simulink model "controlGPI_pos_3dof_conMI"  (R2023b)
settings: Solver=VariableStepAuto  StartTime=0.0  StopTime=tsim  FixedStep=1e-5  MaxStep=tstep  RelTol=1e-3
undefined symbols (not defined in the file): contr_robot_params, ddq, dq, MI_Contr1, MI_Contr2, MI_Contr3, MI_motor1, MI_motor2, MI_motor3, ndof, NN_Bspline_params, NN_RBF_params, nn_select, ns, Pc, q, q0, q_cero, q_eq, robot_params, sigbuilder_block, t_qeq_init, t_tr_init, t_trtr, tau_L, tau_L_mags, tr_muestra, Wc, Zc
libraries: mcbcontrolslib x6, spsRMSLib x6, simulink x2
(part 3 of 3)

== matlab function controlGPI_pos_3dof_conMI/Actuadores (Motores de inducción)/MI1 + PBC Torque Controller/Controlador PBC/Ley de control/Ley de control ==
  data: MI_motor_params input; i_Sref input size=[2,1]; d_iSref input size=[2,1]; U_S output size=[2 1]; psi_Rref input size=[2,1]; w_R input; e_Is input; KI_s input
function U_S = fcn(MI_motor_params,i_Sref,d_iSref,psi_Rref,w_R,e_Is,KI_s)

R_R = MI_motor_params.elecparams.R_R;
L_R = MI_motor_params.elecparams.L_R;
M = MI_motor_params.elecparams.M;
n_p = MI_motor_params.elecparams.n_p;

sigma = MI_motor_params.elecparams.sigma;
gamma = MI_motor_params.elecparams.gamma;

dI_Saref = d_iSref(1);
dI_Sbref = d_iSref(2);

I_Saref = i_Sref(1);
I_Sbref = i_Sref(2);

psi_Raref = psi_Rref(1);
psi_Rbref = psi_Rref(2);

e_ISa = e_Is(1);
e_ISb = e_Is(2);

U_Sa = sigma*dI_Saref - n_p*M/L_R*w_R*psi_Rbref + sigma*gamma*I_Saref - R_R*M/L_R^2*psi_Raref - KI_s*e_ISa;
U_Sb = sigma*dI_Sbref + n_p*M/L_R*w_R*psi_Raref + sigma*gamma*I_Sbref - R_R*M/L_R^2*psi_Rbref - KI_s*e_ISb;

U_S = [U_Sa;U_Sb];

== matlab function controlGPI_pos_3dof_conMI/Actuadores (Motores de inducción)/MI2 + PBC Torque Controller/Modelo MI (Subsistema eléctrico)/Modelo Motor de inducción (Subsistema eléctrico) ==
  data: MI_motor_params input; di_Sab output double size=[2 1]; dpsi_Rab output double size=[2 1]; u_Sab input double size=[2 1]; i_Sab input double size=[2 1]; psi_Rab input double size=[2 1]; w_R input double size=1; tau_R output size=1; tau_L input
function [di_Sab,dpsi_Rab,tau_R] = fcn(MI_motor_params,u_Sab,i_Sab,psi_Rab,w_R,tau_L)

R_S = MI_motor_params.elecparams.R_S;
R_R = MI_motor_params.elecparams.R_R;
L_S = MI_motor_params.elecparams.L_S;
L_R = MI_motor_params.elecparams.L_R;
M = MI_motor_params.elecparams.M;
n_p = MI_motor_params.elecparams.n_p;

J = MI_motor_params.mechparams.J;
b = MI_motor_params.mechparams.b;

sigma = MI_motor_params.elecparams.sigma;
gamma = MI_motor_params.elecparams.gamma;

u_sa = u_Sab(1);
u_sb = u_Sab(2);

i_sa = i_Sab(1);
i_sb = i_Sab(2);

psi_ra = psi_Rab(1);
psi_rb = psi_Rab(2);

tau_R = n_p*M/L_R*(i_sb*psi_ra-i_sa*psi_rb);

x = [i_sa;i_sb;psi_ra;psi_rb];

A = [-gamma      , 0            , (M*R_R)/(sigma*L_R^2)    , (n_p*M)/(sigma*L_R)*w_R ;
     0           , -gamma       , -(n_p*M)/(sigma*L_R)*w_R , (M*R_R)/(sigma*L_R^2)   ; 
     (R_R*M)/L_R , 0            , -R_R/L_R                 , -n_p*w_R                ;
     0           , (R_R*M)/L_R  , n_p*w_R                  , -R_R/L_R                ];

B = [1/sigma , 0       ;
     0       , 1/sigma ;
     0       , 0       ;
     0       , 0       ];

dx = A*x + B*[u_sa;u_sb];

di_Sab = dx(1:2);
dpsi_Rab = dx(3:4);

%Subsistema mecanico
%dw_R = (1/J)*tau_R - (b/J)*w_R - (1/J)*tau_L;

== matlab function controlGPI_pos_3dof_conMI/ControladorGPI + NN/Matriz D ==
  data: robot_params input Bus: robot_params_bus; robot_din output Bus: robot_din_bus; q input
function robot_din = fcn(robot_params,q)

robot_din = robot_dinm.din_3dof(robot_params,q,zeros(size(q)));

== matlab function controlGPI_pos_3dof_conMI/Perfil torque de carga tau_L/If Action Subsystem/Polinomio 7mo orden sen ==
  data: t input; perfil_params input; qpol output; vpol output; apol output; jpol output
function [qpol,vpol,apol,jpol] = fcn(t,perfil_params)

%Trayectoria de referencia

q0 = 0;
q1 = perfil_params.senoidal.amplitud;

% v0 = perfil_params.polinomio7.vel.inicial;
% v1 = perfil_params.polinomio7.vel.final;
% 
% ac0 = perfil_params.polinomio7.acel.inicial;
% ac1 = perfil_params.polinomio7.acel.final;
% 
% j0 = perfil_params.polinomio7.jerk.inicial;
% j1 = perfil_params.polinomio7.jerk.inicial;

if perfil_params.senoidal.tiempo_inicio-1>0
    t0 = perfil_params.senoidal.tiempo_inicio-1;
else
    t0 = 0;
end
t1 = perfil_params.senoidal.tiempo_inicio;

% Coeficientes de un polinomio de 7mo grado
[qpol,vpol,apol,jpol] = pol7(t,q1,q0,t0,t1);

== matlab function controlGPI_pos_3dof_conMI/Perfil torque de carga tau_L/If Action Subsystem/Senoidal tiempo de inicio ==
  data: t input; tr output; perfil_params input
function tr = fcn(t,perfil_params)

t1 = perfil_params.senoidal.tiempo_inicio;

if t < t1
    tr = 0;
else
    tr = t - t1;
end

== matlab function controlGPI_pos_3dof_conMI/Perfil torque de carga tau_L/If Action Subsystem4/Polinomio 7mo orden tau_L ==
  data: t input; perfil_params input; qpol output; vpol output; apol output; jpol output
function [qpol,vpol,apol,jpol] = fcn(t,perfil_params)

%Trayectoria de referencia

q0 = perfil_params.polinomio7.pos.inicial;
q1 = perfil_params.polinomio7.pos.final;

% v0 = perfil_params.polinomio7.vel.inicial;
% v1 = perfil_params.polinomio7.vel.final;
% 
% ac0 = perfil_params.polinomio7.acel.inicial;
% ac1 = perfil_params.polinomio7.acel.final;
% 
% j0 = perfil_params.polinomio7.jerk.inicial;
% j1 = perfil_params.polinomio7.jerk.inicial;

t0 = perfil_params.polinomio7.tiempo.inicial;
t1 = perfil_params.polinomio7.tiempo.final;

% Coeficientes de un polinomio de 7mo grado
[qpol,vpol,apol,jpol] = pol7(t,q0,q1,t0,t1);

== matlab function controlGPI_pos_3dof_conMI/Actuadores (Motores de inducción)/MI2 + PBC Torque Controller/Modelo MI (Subsistema eléctrico)/ab//dq ==
  data: psi_ra input; psi_Rmag output; psi_rb input; rho output
function [psi_Rmag,rho] = fcn(psi_ra,psi_rb)

psi_Rmag = sqrt(psi_ra^2+psi_rb^2);
rho = atan2(psi_rb,psi_ra);

== matlab function controlGPI_pos_3dof_conMI/Perfil torque de carga tau_L/If Action Subsystem5/Tren de esca ==
  data: t input; q output; perfil_params input
function q = fcn(t,perfil_params)

q = Perfil_trayectoria.trEsca(t,perfil_params);

== matlab function controlGPI_pos_3dof_conMI/Perfil torque de carga tau_L/If Action Subsystem6/Polinomio 7mo orden timeseries ==
  data: t input; qpol output; vpol output; apol output; jpol output
function [qpol,vpol,apol,jpol] = fcn(t)

q0 = 0;
q1 = 1;

t0 = 0.5;
t1 = 1;

%Trayectoria de referencia

% Coeficientes de un polinomio de 7mo grado
[qpol,vpol,apol,jpol] = pol7(t,q0,q1,t0,t1);

== matlab function controlGPI_pos_3dof_conMI/Perfil torque de carga tau_L/If Action Subsystem7/Trayectoria 15 segmentos ==
  data: t input size=1; q output size=1; perfil_params input
function q = fcn(t,perfil_params)

q0 = perfil_params.tr15segs.pos.inicial;
q1 = perfil_params.tr15segs.pos.final;

t0 = perfil_params.tr15segs.tiempo.inicial;

vel_path = perfil_params.tr15segs.vel_path;
acel_path = perfil_params.tr15segs.acel_path;
snap_path = perfil_params.tr15segs.snap_path;

dist = norm(q1-q0);
num_steps = 1000;




[interq,T] = pol15segs.bounded_tr(dist,num_steps,vel_path,acel_path,snap_path,0);

tstep = T/num_steps;
t1 = t0 + T;
t_tr = (t0:tstep:t1)';


[~,idt] = min(t_tr-t);
dire = (q1 - q0)/dist;
q = q0 + dire*interq(idt);

== matlab function controlGPI_pos_3dof_conMI/Modelo robot manipulador (Dinámica directa)/Dinámica directa ==
  data: robot_params input; q input; ddq output size=[3,1]; dq input size=[3,1]; tau_R input size=[3,1]; tau_L input size=[3,1]
function ddq = fcn(robot_params,q,dq,tau_R,tau_L)

robot_din = robot_dinm.din_3dof(robot_params,q,dq);

D = robot_din.D;
C = robot_din.C;
G = robot_din.G;
g = robot_din.g;

ddq = D^-1*(-C*dq-G*g+(tau_R-tau_L));

== matlab function controlGPI_pos_3dof_conMI/Actuadores (Motores de inducción)/MI1 + PBC Torque Controller/Controlador PBC/Corrientes y Flujos deseados/Corrientes//Flujos deseados ==
  data: MI_motor_params input; w_R input; i_Sref output size=[2 1]; psi_Rref input size=[2,1]; tau_Rref input; psi_Rmagref input; dpsi_Rmagref input; dpsi_Rref output size=[2,1]
function [i_Sref,dpsi_Rref] = fcn(MI_motor_params,w_R,psi_Rref,tau_Rref,psi_Rmagref,dpsi_Rmagref)

R_R = MI_motor_params.elecparams.R_R;
L_R = MI_motor_params.elecparams.L_R;
M = MI_motor_params.elecparams.M;
n_p = MI_motor_params.elecparams.n_p;

psi_Raref = psi_Rref(1);
psi_Rbref = psi_Rref(2);

i_Saref =  - L_R/(M*n_p*psi_Rmagref^2)*tau_Rref*psi_Rbref + 1/M*psi_Raref + L_R/(R_R*M)*dpsi_Rmagref/psi_Rmagref*psi_Raref;
i_Sbref =  + L_R/(M*n_p*psi_Rmagref^2)*tau_Rref*psi_Raref + 1/M*psi_Rbref + L_R/(R_R*M)*dpsi_Rmagref/psi_Rmagref*psi_Rbref;

i_Sref = [i_Saref;i_Sbref];

dpsi_Raref = - (n_p*w_R + R_R/(n_p*psi_Rmagref^2)*tau_Rref)*psi_Rbref + dpsi_Rmagref/psi_Rmagref*psi_Raref;
dpsi_Rbref = + (n_p*w_R + R_R/(n_p*psi_Rmagref^2)*tau_Rref)*psi_Raref + dpsi_Rmagref/psi_Rmagref*psi_Rbref;

dpsi_Rref = [dpsi_Raref;dpsi_Rbref];

== matlab function controlGPI_pos_3dof_conMI/Actuadores (Motores de inducción)/MI1 + PBC Torque Controller/Controlador PBC/Ley de control/K_iS ==
  data: MI_motor_params input; w_R input; epsilon input; K_iS output
function K_iS = fcn(MI_motor_params,w_R,epsilon)

R_R = MI_motor_params.elecparams.R_R;
M = MI_motor_params.elecparams.M;
L_R = MI_motor_params.elecparams.L_R;
n_p = MI_motor_params.elecparams.n_p;


K_iS = M^2*L_R*n_p^2*w_R^2/(epsilon*4*R_R);

== matlab function controlGPI_pos_3dof_conMI/Actuadores (Motores de inducción)/MI1 + PBC Torque Controller/Calculo de Potencia eléctrica/ab0 - ABC ==
  data: BPU input size=[2,1]; U output size=[3,1]
function U = fcn(BPU)

BPU = vertcat(BPU,0);

% BP = 2/3*[1,-1/2,-1/2;
%           0,sqrt(3)/2,-sqrt(3)/2;
%           1/2,1/2,1/2];

% Power invariant
BP = sqrt(2/3)*[1,-1/2,-1/2;
                0,sqrt(3)/2,-sqrt(3)/2
                1/sqrt(2),1/sqrt(2),1/sqrt(2)];

U = BP^-1*BPU;

== matlab function controlGPI_pos_3dof_conMI/Actuadores (Motores de inducción)/MI1 + PBC Torque Controller/Calculo de Potencia eléctrica/ab0 - ABC1 ==
  data: BPU input size=[2,1]; U output size=[3,1]
function U = fcn(BPU)

BPU = vertcat(BPU,0);

% BP = 2/3*[1,-1/2,-1/2;
%           0,sqrt(3)/2,-sqrt(3)/2;
%           1/2,1/2,1/2];

% Power invariant
BP = sqrt(2/3)*[1,-1/2,-1/2;
                0,sqrt(3)/2,-sqrt(3)/2
                1/sqrt(2),1/sqrt(2),1/sqrt(2)];

U = BP^-1*BPU;

== matlab function controlGPI_pos_3dof_conMI/Actuadores (Motores de inducción)/MI2 + PBC Torque Controller/Calculo de Potencia eléctrica/ab0 - ABC ==
  data: BPU input size=[2,1]; U output size=[3,1]
function U = fcn(BPU)

BPU = vertcat(BPU,0);

% BP = 2/3*[1,-1/2,-1/2;
%           0,sqrt(3)/2,-sqrt(3)/2;
%           1/2,1/2,1/2];

% Power invariant
BP = sqrt(2/3)*[1,-1/2,-1/2;
                0,sqrt(3)/2,-sqrt(3)/2
                1/sqrt(2),1/sqrt(2),1/sqrt(2)];

U = BP^-1*BPU;

== matlab function controlGPI_pos_3dof_conMI/Actuadores (Motores de inducción)/MI2 + PBC Torque Controller/Calculo de Potencia eléctrica/ab0 - ABC1 ==
  data: BPU input size=[2,1]; U output size=[3,1]
function U = fcn(BPU)

BPU = vertcat(BPU,0);

% BP = 2/3*[1,-1/2,-1/2;
%           0,sqrt(3)/2,-sqrt(3)/2;
%           1/2,1/2,1/2];

% Power invariant
BP = sqrt(2/3)*[1,-1/2,-1/2;
                0,sqrt(3)/2,-sqrt(3)/2
                1/sqrt(2),1/sqrt(2),1/sqrt(2)];

U = BP^-1*BPU;

== matlab function controlGPI_pos_3dof_conMI/Actuadores (Motores de inducción)/MI2 + PBC Torque Controller/Controlador PBC/Corrientes y Flujos deseados/Corrientes//Flujos deseados ==
  data: MI_motor_params input; w_R input; i_Sref output size=[2 1]; psi_Rref input size=[2,1]; tau_Rref input; psi_Rmagref input; dpsi_Rmagref input; dpsi_Rref output size=[2,1]
function [i_Sref,dpsi_Rref] = fcn(MI_motor_params,w_R,psi_Rref,tau_Rref,psi_Rmagref,dpsi_Rmagref)

R_R = MI_motor_params.elecparams.R_R;
L_R = MI_motor_params.elecparams.L_R;
M = MI_motor_params.elecparams.M;
n_p = MI_motor_params.elecparams.n_p;

psi_Raref = psi_Rref(1);
psi_Rbref = psi_Rref(2);

i_Saref =  - L_R/(M*n_p*psi_Rmagref^2)*tau_Rref*psi_Rbref + 1/M*psi_Raref + L_R/(R_R*M)*dpsi_Rmagref/psi_Rmagref*psi_Raref;
i_Sbref =  + L_R/(M*n_p*psi_Rmagref^2)*tau_Rref*psi_Raref + 1/M*psi_Rbref + L_R/(R_R*M)*dpsi_Rmagref/psi_Rmagref*psi_Rbref;

i_Sref = [i_Saref;i_Sbref];

dpsi_Raref = - (n_p*w_R + R_R/(n_p*psi_Rmagref^2)*tau_Rref)*psi_Rbref + dpsi_Rmagref/psi_Rmagref*psi_Raref;
dpsi_Rbref = + (n_p*w_R + R_R/(n_p*psi_Rmagref^2)*tau_Rref)*psi_Raref + dpsi_Rmagref/psi_Rmagref*psi_Rbref;

dpsi_Rref = [dpsi_Raref;dpsi_Rbref];

== matlab function controlGPI_pos_3dof_conMI/Actuadores (Motores de inducción)/MI1 + PBC Torque Controller/Controlador PBC/derivada Corrientes deseadas/derivada Corrientes deseadas ==
  data: MI_motor_params input; d_iSref output size=[2 1]; psi_Rref input size=[2,1]; dpsi_Rref input size=[2,1]; psi_Rmagref input; dpsi_Rmagref input; ddpsi_Rmagref input; tau_Rref input; dtau_Rref input
function d_iSref = fcn(MI_motor_params,psi_Rref,dpsi_Rref,psi_Rmagref,dpsi_Rmagref,ddpsi_Rmagref,tau_Rref,dtau_Rref)

R_R = MI_motor_params.elecparams.R_R;
L_R = MI_motor_params.elecparams.L_R;
M = MI_motor_params.elecparams.M;
n_p = MI_motor_params.elecparams.n_p;

dpsi_Raref = dpsi_Rref(1);
dpsi_Rbref = dpsi_Rref(2);

psi_Raref = psi_Rref(1);
psi_Rbref = psi_Rref(2);

dI_Saref = L_R/(M*n_p)*(- ((dtau_Rref-2*tau_Rref*dpsi_Rmagref)/psi_Rmagref)*psi_Rbref - tau_Rref/psi_Rmagref^2*dpsi_Rbref) + dpsi_Raref/M ...
         + L_R/(R_R*M)*(((ddpsi_Rmagref*psi_Rmagref-dpsi_Rmagref^2)/psi_Rmagref^2)*psi_Raref + dpsi_Rmagref/psi_Rmagref*dpsi_Raref);

dI_Sbref = L_R/(M*n_p)*(+ ((dtau_Rref-2*tau_Rref*dpsi_Rmagref)/psi_Rmagref)*psi_Raref + tau_Rref/psi_Rmagref^2*dpsi_Raref) + dpsi_Rbref/M ...
         + L_R/(R_R*M)*(((ddpsi_Rmagref*psi_Rmagref-dpsi_Rmagref^2)/psi_Rmagref^2)*psi_Rbref + dpsi_Rmagref/psi_Rmagref*dpsi_Rbref);

d_iSref = [dI_Saref;dI_Sbref];

== matlab function controlGPI_pos_3dof_conMI/Actuadores (Motores de inducción)/MI1 + PBC Torque Controller/Modelo MI (Subsistema eléctrico)/Modelo Motor de inducción (Subsistema eléctrico) ==
  data: MI_motor_params input; di_Sab output double size=[2 1]; dpsi_Rab output double size=[2 1]; u_Sab input double size=[2 1]; i_Sab input double size=[2 1]; psi_Rab input double size=[2 1]; w_R input double size=1; tau_R output size=1; tau_L input
function [di_Sab,dpsi_Rab,tau_R] = fcn(MI_motor_params,u_Sab,i_Sab,psi_Rab,w_R,tau_L)

R_S = MI_motor_params.elecparams.R_S;
R_R = MI_motor_params.elecparams.R_R;
L_S = MI_motor_params.elecparams.L_S;
L_R = MI_motor_params.elecparams.L_R;
M = MI_motor_params.elecparams.M;
n_p = MI_motor_params.elecparams.n_p;

J = MI_motor_params.mechparams.J;
b = MI_motor_params.mechparams.b;

sigma = MI_motor_params.elecparams.sigma;
gamma = MI_motor_params.elecparams.gamma;

u_sa = u_Sab(1);
u_sb = u_Sab(2);

i_sa = i_Sab(1);
i_sb = i_Sab(2);

psi_ra = psi_Rab(1);
psi_rb = psi_Rab(2);

tau_R = n_p*M/L_R*(i_sb*psi_ra-i_sa*psi_rb);

x = [i_sa;i_sb;psi_ra;psi_rb];

A = [-gamma      , 0            , (M*R_R)/(sigma*L_R^2)    , (n_p*M)/(sigma*L_R)*w_R ;
     0           , -gamma       , -(n_p*M)/(sigma*L_R)*w_R , (M*R_R)/(sigma*L_R^2)   ; 
     (R_R*M)/L_R , 0            , -R_R/L_R                 , -n_p*w_R                ;
     0           , (R_R*M)/L_R  , n_p*w_R                  , -R_R/L_R                ];

B = [1/sigma , 0       ;
     0       , 1/sigma ;
     0       , 0       ;
     0       , 0       ];

dx = A*x + B*[u_sa;u_sb];

di_Sab = dx(1:2);
dpsi_Rab = dx(3:4);

%Subsistema mecanico
%dw_R = (1/J)*tau_R - (b/J)*w_R - (1/J)*tau_L;

== matlab function controlGPI_pos_3dof_conMI/Norm e_q ==
  data: u input; y output
function y = norm(u)

y = norm(u,2);

== matlab function controlGPI_pos_3dof_conMI/Actuadores (Motores de inducción)/MI1 + PBC Torque Controller/Modelo MI (Subsistema eléctrico)/ab//dq ==
  data: psi_ra input; psi_Rmag output; psi_rb input; rho output
function [psi_Rmag,rho] = fcn(psi_ra,psi_rb)

psi_Rmag = sqrt(psi_ra^2+psi_rb^2);
rho = atan2(psi_rb,psi_ra);

== matlab function controlGPI_pos_3dof_conMI/Actuadores (Motores de inducción)/MI2 + PBC Torque Controller/Controlador PBC/Ley de control/K_iS ==
  data: MI_motor_params input; w_R input; epsilon input; K_iS output
function K_iS = fcn(MI_motor_params,w_R,epsilon)

R_R = MI_motor_params.elecparams.R_R;
M = MI_motor_params.elecparams.M;
L_R = MI_motor_params.elecparams.L_R;
n_p = MI_motor_params.elecparams.n_p;


K_iS = M^2*L_R*n_p^2*w_R^2/(epsilon*4*R_R);

== matlab function controlGPI_pos_3dof_conMI/Actuadores (Motores de inducción)/MI2 + PBC Torque Controller/Controlador PBC/Ley de control/Ley de control ==
  data: MI_motor_params input; i_Sref input size=[2,1]; d_iSref input size=[2,1]; U_S output size=[2 1]; psi_Rref input size=[2,1]; w_R input; e_Is input; KI_s input
function U_S = fcn(MI_motor_params,i_Sref,d_iSref,psi_Rref,w_R,e_Is,KI_s)

R_R = MI_motor_params.elecparams.R_R;
L_R = MI_motor_params.elecparams.L_R;
M = MI_motor_params.elecparams.M;
n_p = MI_motor_params.elecparams.n_p;

sigma = MI_motor_params.elecparams.sigma;
gamma = MI_motor_params.elecparams.gamma;

dI_Saref = d_iSref(1);
dI_Sbref = d_iSref(2);

I_Saref = i_Sref(1);
I_Sbref = i_Sref(2);

psi_Raref = psi_Rref(1);
psi_Rbref = psi_Rref(2);

e_ISa = e_Is(1);
e_ISb = e_Is(2);

U_Sa = sigma*dI_Saref - n_p*M/L_R*w_R*psi_Rbref + sigma*gamma*I_Saref - R_R*M/L_R^2*psi_Raref - KI_s*e_ISa;
U_Sb = sigma*dI_Sbref + n_p*M/L_R*w_R*psi_Raref + sigma*gamma*I_Sbref - R_R*M/L_R^2*psi_Rbref - KI_s*e_ISb;

U_S = [U_Sa;U_Sb];

== matlab function controlGPI_pos_3dof_conMI/Actuadores (Motores de inducción)/MI2 + PBC Torque Controller/Controlador PBC/derivada Corrientes deseadas/derivada Corrientes deseadas ==
  data: MI_motor_params input; d_iSref output size=[2 1]; psi_Rref input size=[2,1]; dpsi_Rref input size=[2,1]; psi_Rmagref input; dpsi_Rmagref input; ddpsi_Rmagref input; tau_Rref input; dtau_Rref input
function d_iSref = fcn(MI_motor_params,psi_Rref,dpsi_Rref,psi_Rmagref,dpsi_Rmagref,ddpsi_Rmagref,tau_Rref,dtau_Rref)

R_R = MI_motor_params.elecparams.R_R;
L_R = MI_motor_params.elecparams.L_R;
M = MI_motor_params.elecparams.M;
n_p = MI_motor_params.elecparams.n_p;

dpsi_Raref = dpsi_Rref(1);
dpsi_Rbref = dpsi_Rref(2);

psi_Raref = psi_Rref(1);
psi_Rbref = psi_Rref(2);

dI_Saref = L_R/(M*n_p)*(- ((dtau_Rref-2*tau_Rref*dpsi_Rmagref)/psi_Rmagref)*psi_Rbref - tau_Rref/psi_Rmagref^2*dpsi_Rbref) + dpsi_Raref/M ...
         + L_R/(R_R*M)*(((ddpsi_Rmagref*psi_Rmagref-dpsi_Rmagref^2)/psi_Rmagref^2)*psi_Raref + dpsi_Rmagref/psi_Rmagref*dpsi_Raref);

dI_Sbref = L_R/(M*n_p)*(+ ((dtau_Rref-2*tau_Rref*dpsi_Rmagref)/psi_Rmagref)*psi_Raref + tau_Rref/psi_Rmagref^2*dpsi_Raref) + dpsi_Rbref/M ...
         + L_R/(R_R*M)*(((ddpsi_Rmagref*psi_Rmagref-dpsi_Rmagref^2)/psi_Rmagref^2)*psi_Rbref + dpsi_Rmagref/psi_Rmagref*dpsi_Rbref);

d_iSref = [dI_Saref;dI_Sbref];

== matlab function controlGPI_pos_3dof_conMI/Actuadores (Motores de inducción)/MI3 + PBC Torque Controller/Calculo de Potencia eléctrica/ab0 - ABC ==
  data: BPU input size=[2,1]; U output size=[3,1]
function U = fcn(BPU)

BPU = vertcat(BPU,0);

% BP = 2/3*[1,-1/2,-1/2;
%           0,sqrt(3)/2,-sqrt(3)/2;
%           1/2,1/2,1/2];

% Power invariant
BP = sqrt(2/3)*[1,-1/2,-1/2;
                0,sqrt(3)/2,-sqrt(3)/2
                1/sqrt(2),1/sqrt(2),1/sqrt(2)];

U = BP^-1*BPU;

== matlab function controlGPI_pos_3dof_conMI/Actuadores (Motores de inducción)/MI3 + PBC Torque Controller/Calculo de Potencia eléctrica/ab0 - ABC1 ==
  data: BPU input size=[2,1]; U output size=[3,1]
function U = fcn(BPU)

BPU = vertcat(BPU,0);

% BP = 2/3*[1,-1/2,-1/2;
%           0,sqrt(3)/2,-sqrt(3)/2;
%           1/2,1/2,1/2];

% Power invariant
BP = sqrt(2/3)*[1,-1/2,-1/2;
                0,sqrt(3)/2,-sqrt(3)/2
                1/sqrt(2),1/sqrt(2),1/sqrt(2)];

U = BP^-1*BPU;

== matlab function controlGPI_pos_3dof_conMI/Actuadores (Motores de inducción)/MI3 + PBC Torque Controller/Controlador PBC/Corrientes y Flujos deseados/Corrientes//Flujos deseados ==
  data: MI_motor_params input; w_R input; i_Sref output size=[2 1]; psi_Rref input size=[2,1]; tau_Rref input; psi_Rmagref input; dpsi_Rmagref input; dpsi_Rref output size=[2,1]
function [i_Sref,dpsi_Rref] = fcn(MI_motor_params,w_R,psi_Rref,tau_Rref,psi_Rmagref,dpsi_Rmagref)

R_R = MI_motor_params.elecparams.R_R;
L_R = MI_motor_params.elecparams.L_R;
M = MI_motor_params.elecparams.M;
n_p = MI_motor_params.elecparams.n_p;

psi_Raref = psi_Rref(1);
psi_Rbref = psi_Rref(2);

i_Saref =  - L_R/(M*n_p*psi_Rmagref^2)*tau_Rref*psi_Rbref + 1/M*psi_Raref + L_R/(R_R*M)*dpsi_Rmagref/psi_Rmagref*psi_Raref;
i_Sbref =  + L_R/(M*n_p*psi_Rmagref^2)*tau_Rref*psi_Raref + 1/M*psi_Rbref + L_R/(R_R*M)*dpsi_Rmagref/psi_Rmagref*psi_Rbref;

i_Sref = [i_Saref;i_Sbref];

dpsi_Raref = - (n_p*w_R + R_R/(n_p*psi_Rmagref^2)*tau_Rref)*psi_Rbref + dpsi_Rmagref/psi_Rmagref*psi_Raref;
dpsi_Rbref = + (n_p*w_R + R_R/(n_p*psi_Rmagref^2)*tau_Rref)*psi_Raref + dpsi_Rmagref/psi_Rmagref*psi_Rbref;

dpsi_Rref = [dpsi_Raref;dpsi_Rbref];

== matlab function controlGPI_pos_3dof_conMI/Trayectoria de referencia/Dinamica inversa (referencia) ==
  data: robot_params input; tau_s output size=[3,1]; q input size=[3,1]; dq input size=[3,1]; ddq input size=[3,1]
function tau_s = fcn(robot_params,q,dq,ddq)

robot_din = robot_dinm.din_3dof(robot_params,q,dq);

D = robot_din.D;
C = robot_din.C;
G = robot_din.G;
g = robot_din.g;

tau_s = D*ddq + C*dq + G*g;

== matlab function controlGPI_pos_3dof_conMI/Actuadores (Motores de inducción)/MI3 + PBC Torque Controller/Controlador PBC/Ley de control/K_iS ==
  data: MI_motor_params input; w_R input; epsilon input; K_iS output
function K_iS = fcn(MI_motor_params,w_R,epsilon)

R_R = MI_motor_params.elecparams.R_R;
M = MI_motor_params.elecparams.M;
L_R = MI_motor_params.elecparams.L_R;
n_p = MI_motor_params.elecparams.n_p;


K_iS = M^2*L_R*n_p^2*w_R^2/(epsilon*4*R_R);

== matlab function controlGPI_pos_3dof_conMI/Actuadores (Motores de inducción)/MI3 + PBC Torque Controller/Controlador PBC/Ley de control/Ley de control ==
  data: MI_motor_params input; i_Sref input size=[2,1]; d_iSref input size=[2,1]; U_S output size=[2 1]; psi_Rref input size=[2,1]; w_R input; e_Is input; KI_s input
function U_S = fcn(MI_motor_params,i_Sref,d_iSref,psi_Rref,w_R,e_Is,KI_s)

R_R = MI_motor_params.elecparams.R_R;
L_R = MI_motor_params.elecparams.L_R;
M = MI_motor_params.elecparams.M;
n_p = MI_motor_params.elecparams.n_p;

sigma = MI_motor_params.elecparams.sigma;
gamma = MI_motor_params.elecparams.gamma;

dI_Saref = d_iSref(1);
dI_Sbref = d_iSref(2);

I_Saref = i_Sref(1);
I_Sbref = i_Sref(2);

psi_Raref = psi_Rref(1);
psi_Rbref = psi_Rref(2);

e_ISa = e_Is(1);
e_ISb = e_Is(2);

U_Sa = sigma*dI_Saref - n_p*M/L_R*w_R*psi_Rbref + sigma*gamma*I_Saref - R_R*M/L_R^2*psi_Raref - KI_s*e_ISa;
U_Sb = sigma*dI_Sbref + n_p*M/L_R*w_R*psi_Raref + sigma*gamma*I_Sbref - R_R*M/L_R^2*psi_Rbref - KI_s*e_ISb;

U_S = [U_Sa;U_Sb];

== matlab function controlGPI_pos_3dof_conMI/Actuadores (Motores de inducción)/MI3 + PBC Torque Controller/Controlador PBC/derivada Corrientes deseadas/derivada Corrientes deseadas ==
  data: MI_motor_params input; d_iSref output size=[2 1]; psi_Rref input size=[2,1]; dpsi_Rref input size=[2,1]; psi_Rmagref input; dpsi_Rmagref input; ddpsi_Rmagref input; tau_Rref input; dtau_Rref input
function d_iSref = fcn(MI_motor_params,psi_Rref,dpsi_Rref,psi_Rmagref,dpsi_Rmagref,ddpsi_Rmagref,tau_Rref,dtau_Rref)

R_R = MI_motor_params.elecparams.R_R;
L_R = MI_motor_params.elecparams.L_R;
M = MI_motor_params.elecparams.M;
n_p = MI_motor_params.elecparams.n_p;

dpsi_Raref = dpsi_Rref(1);
dpsi_Rbref = dpsi_Rref(2);

psi_Raref = psi_Rref(1);
psi_Rbref = psi_Rref(2);

dI_Saref = L_R/(M*n_p)*(- ((dtau_Rref-2*tau_Rref*dpsi_Rmagref)/psi_Rmagref)*psi_Rbref - tau_Rref/psi_Rmagref^2*dpsi_Rbref) + dpsi_Raref/M ...
         + L_R/(R_R*M)*(((ddpsi_Rmagref*psi_Rmagref-dpsi_Rmagref^2)/psi_Rmagref^2)*psi_Raref + dpsi_Rmagref/psi_Rmagref*dpsi_Raref);

dI_Sbref = L_R/(M*n_p)*(+ ((dtau_Rref-2*tau_Rref*dpsi_Rmagref)/psi_Rmagref)*psi_Raref + tau_Rref/psi_Rmagref^2*dpsi_Raref) + dpsi_Rbref/M ...
         + L_R/(R_R*M)*(((ddpsi_Rmagref*psi_Rmagref-dpsi_Rmagref^2)/psi_Rmagref^2)*psi_Rbref + dpsi_Rmagref/psi_Rmagref*dpsi_Rbref);

d_iSref = [dI_Saref;dI_Sbref];

== matlab function controlGPI_pos_3dof_conMI/Actuadores (Motores de inducción)/MI3 + PBC Torque Controller/Modelo MI (Subsistema eléctrico)/Modelo Motor de inducción (Subsistema eléctrico) ==
  data: MI_motor_params input; di_Sab output double size=[2 1]; dpsi_Rab output double size=[2 1]; u_Sab input double size=[2 1]; i_Sab input double size=[2 1]; psi_Rab input double size=[2 1]; w_R input double size=1; tau_R output size=1; tau_L input
function [di_Sab,dpsi_Rab,tau_R] = fcn(MI_motor_params,u_Sab,i_Sab,psi_Rab,w_R,tau_L)

R_S = MI_motor_params.elecparams.R_S;
R_R = MI_motor_params.elecparams.R_R;
L_S = MI_motor_params.elecparams.L_S;
L_R = MI_motor_params.elecparams.L_R;
M = MI_motor_params.elecparams.M;
n_p = MI_motor_params.elecparams.n_p;

J = MI_motor_params.mechparams.J;
b = MI_motor_params.mechparams.b;

sigma = MI_motor_params.elecparams.sigma;
gamma = MI_motor_params.elecparams.gamma;

u_sa = u_Sab(1);
u_sb = u_Sab(2);

i_sa = i_Sab(1);
i_sb = i_Sab(2);

psi_ra = psi_Rab(1);
psi_rb = psi_Rab(2);

tau_R = n_p*M/L_R*(i_sb*psi_ra-i_sa*psi_rb);

x = [i_sa;i_sb;psi_ra;psi_rb];

A = [-gamma      , 0            , (M*R_R)/(sigma*L_R^2)    , (n_p*M)/(sigma*L_R)*w_R ;
     0           , -gamma       , -(n_p*M)/(sigma*L_R)*w_R , (M*R_R)/(sigma*L_R^2)   ; 
     (R_R*M)/L_R , 0            , -R_R/L_R                 , -n_p*w_R                ;
     0           , (R_R*M)/L_R  , n_p*w_R                  , -R_R/L_R                ];

B = [1/sigma , 0       ;
     0       , 1/sigma ;
     0       , 0       ;
     0       , 0       ];

dx = A*x + B*[u_sa;u_sb];

di_Sab = dx(1:2);
dpsi_Rab = dx(3:4);

%Subsistema mecanico
%dw_R = (1/J)*tau_R - (b/J)*w_R - (1/J)*tau_L;

== matlab function controlGPI_pos_3dof_conMI/Actuadores (Motores de inducción)/MI3 + PBC Torque Controller/Modelo MI (Subsistema eléctrico)/ab//dq ==
  data: psi_ra input; psi_Rmag output; psi_rb input; rho output
function [psi_Rmag,rho] = fcn(psi_ra,psi_rb)

psi_Rmag = sqrt(psi_ra^2+psi_rb^2);
rho = atan2(psi_rb,psi_ra);

== matlab function controlGPI_pos_3dof_conMI/ControladorGPI + NN/Ley de control ==
  data: robot_din input; v output size=[3,1]; eqB5 input size=[3,1]; eqB4 input size=[3,1]; eqB3 input size=[3,1]; eqB2 input size=[3,1]; eqB1 input size=[3,1]; tau_R output size=[3,1]
function [v,tau_R] = fcn(robot_din,eqB5,eqB4,eqB3,eqB2,eqB1)

D = robot_din.D;

v = - eqB5 - eqB4 - eqB3 - eqB2 - eqB1;

tau_R = D*v;

== matlab function controlGPI_pos_3dof_conMI/Trayectoria de referencia/Inicializar posición de robot manipulador/interp_pol7_q_r ==
  data: t input; q_eq input; interp_qpos output; q_cero input; q_tr_init input; t0 input; t1 input; t_trtr input; tr_muestra input; ndof input
function interp_qpos = fcn(t,q_eq,q_cero,q_tr_init,t0,t1,t_trtr,tr_muestra,ndof)

tcero = t0/2 + t1/2;

if t < tcero
    dist1 = norm(zeros(size(q_eq)) - q_eq);
    
    if dist1 > 0
        qpol1 = pol7(t,0,dist1,t0,tcero);
        dire1 = (zeros(size(q_eq)) - q_eq)/dist1;
        
        interp_qpos = q_eq + dire1*qpol1;
    else
        interp_qpos = q_eq;
    end
elseif t >= tcero && t < t1
    dist2 = norm(q_cero - zeros(size(q_eq)));
    if dist2 > 0
        qpol2 = pol7(t,0,dist2,tcero,t1);
        dire2 = (q_cero - zeros(size(q_eq)))/dist2;
    
        interp_qpos =  zeros(size(q_eq)) + dire2*qpol2;
    else
        interp_qpos = zeros(size(q_eq));
    end
elseif t >= t1 && t < t1 + t_trtr
    if (tr_muestra == 1 || ndof ~= 6) && ndof ~= 2
        dist3 = norm(q_tr_init - q_cero);
        if dist3 > 0
            qpol3 = pol7(t,0,dist3,t1,t1 + t_trtr);
            dire3 = (q_tr_init - q_cero)/dist3;
            
            interp_qpos =  q_cero + dire3*qpol3;
        else
            interp_qpos = q_cero;
        end
    else
        interp_qpos = q_tr_init;
    end
elseif t >= t1 + t_trtr
    interp_qpos = q_tr_init;
else
    interp_qpos = q_eq;
end

== matlab function controlGPI_pos_3dof_conMI/ControladorGPI + NN/Matriz de parámetros B ==
  data: B5 output size=[3,1]; B4 output size=[3,1]; B3 output size=[3,1]; B2 output size=[3,1]; Zc input size=[3,1]; B1 output size=[3,1]; Wc input size=[3,1]; Pc input size=[3,1]
function [B5,B4,B3,B2,B1] = fcn(Zc,Wc,Pc)

B = zeros(3,6);

B(:,1) = Wc.^4.*Pc;
B(:,2) = 4*Wc.^3.*Zc.*Pc + Wc.^4;
B(:,3) = 4*Wc.^3.*Zc + 4*Wc.^2.*Zc.^2.*Pc + 2.*Wc.^2.*Pc;
B(:,4) = 2*Wc.^2 + 4*Wc.^2.*Zc.^2 + 4*Wc.*Zc.*Pc;
B(:,5) = 4*Wc.*Zc + Pc;
% B(:,6) = ones(3,6);

B1 = B(:,1);
B2 = B(:,2);
B3 = B(:,3);
B4 = B(:,4);
B5 = B(:,5);
% B6 = B(:,6);

== matlab function controlGPI_pos_3dof_conMI/Trayectoria de referencia/q to xyz (referencia) ==
  data: p output size=[3,3]; robot_params input; q input size=[3,1]
function p = fcn(robot_params,q)

p = robot_cin.cin_dirp_3dof(robot_params,q);
